simulink model "untitled"  (R2023b)
settings: Solver=VariableStepAuto  StartTime=0.0  StopTime=5  FixedStep=0.001  RelTol=1e-3
values from neighbouring files (symbols this model uses):
  i_a_rated = 27    [speed_control_by_field_weakening_parameter.m]
  J = 0.068    [speed_control_by_field_weakening_parameter.m]
  Ka = 1    [speed_control_by_field_weakening_parameter.m]
  La = 2.3e-3    (= 0.0023)    [speed_control_by_field_weakening_parameter.m]
  Ra = 0.3    [speed_control_by_field_weakening_parameter.m]
  speed_base = 2500*2*pi/60    (= 261.799387799)    [speed_control_by_field_weakening_parameter.m]
  speed_ref = 4500    [speed_control_by_field_weakening_parameter.m]
  Tload = 0    [speed_control_by_field_weakening_parameter.m]
  v_t_rated = 230    [speed_control_by_field_weakening_parameter.m]
libraries: slpidlib x2, simulink_extras x1
settings Model: NumberOfSteps=10  Creator=chayutht  LastModifiedBy=chayutht

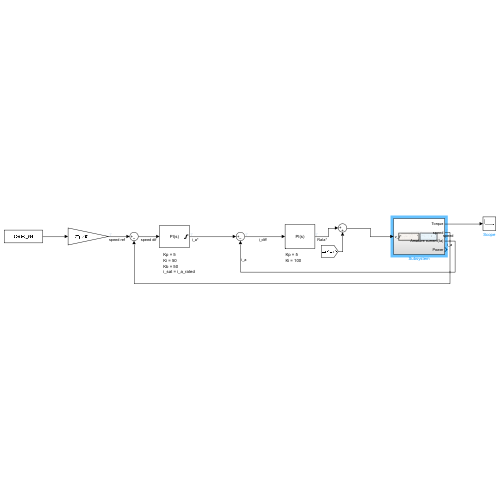
[thumbnail: Simulink's stored preview of the top-level diagram]
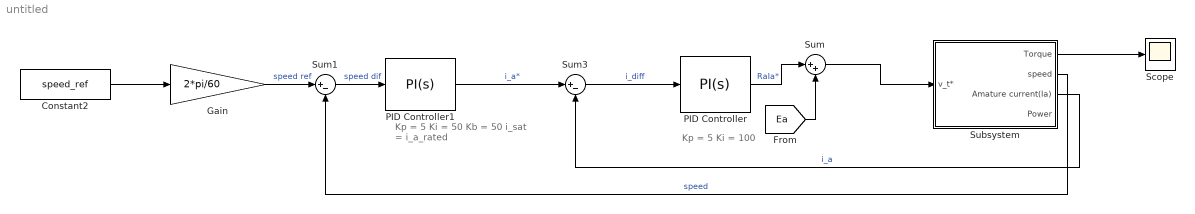
== system untitled ==
  note: Kp = 5
      | Ki = 100
  note: Kp = 5
      | Ki = 50
      | Kb = 50
      | i_sat = i_a_rated
  Constant2 : Constant  Value=speed_ref
  Gain : Gain  Gain=2*pi/60
  PID Controller : slpidlib/PID Controller  Controller=PI  Form=Parallel  TimeDomain=Continuous-time  UseExternalTs=off  SampleTime=-1  IntegratorMethod=Forward Euler  FilterMethod=Forward Euler  ControllerParametersSource=internal  P=5  I=100  UseKiTs=off  D=0.0001  N=100  UseFilter=on  TunerSelectOption=Frequency Response Based  InitialConditionSource=internal  InitialConditionForIntegrator=0  InitialConditionForFilter=0  DifferentiatorICPrevScaledInput=0  ExternalReset=none  TrackingMode=off  Kt=1  LimitOutput=off  SatLimitsSource=internal  UpperSaturationLimit=v_t_rated  LowerSaturationLimit=0  LinearizeAsGain=on  AntiWindupMode=none  Kb=1  LimitIntegrator=off  UpperIntegratorSaturationLimit=inf  LowerIntegratorSaturationLimit=-inf  POutMin=[]  POutMax=[]  IOutMin=[]  IOutMax=[]  DOutMin=[]  DOutMax=[]  NOutMin=[]  NOutMax=[]  SumOutMin=[]  SumOutMax=[]  SaturationOutMin=[]  SaturationOutMax=[]  PParamMin=[]  PParamMax=[]  IParamMin=[]  IParamMax=[]  DParamMin=[]  DParamMax=[]  NParamMin=[]  NParamMax=[]  KbParamMin=[]  KbParamMax=[]  KtParamMin=[]  KtParamMax=[]  KbOutMin=[]  KbOutMax=[]  KtOutMin=[]  KtOutMax=[]  IntegratorOutMin=[]  IntegratorOutMax=[]  FilterOutMin=[]  FilterOutMax=[]  SumI1OutMin=[]  SumI1OutMax=[]  SumI2OutMin=[]  SumI2OutMax=[]  SumI3OutMin=[]  SumI3OutMax=[]  SumI4OutMin=[]  SumI4OutMax=[]  SumDOutMin=[]  SumDOutMax=[]  DifferentiatorOutMin=[]  DifferentiatorOutMax=[]  FilterDiffOutCoefMin=[]  FilterDiffOutCoefMax=[]  ReciprocalOutMin=[]  ReciprocalOutMax=[]  SumDenOutMin=[]  SumDenOutMax=[]  SumNumOutMin=[]  SumNumOutMax=[]  DivideOutMin=[]  DivideOutMax=[]  UdiffTsProdOutMin=[]  UdiffTsProdOutMax=[]  NTsProdOutMin=[]  NTsProdOutMax=[]  UintegralTsProdOutMin=[]  UintegralTsProdOutMax=[]  UngainTsProdOutMin=[]  UngainTsProdOutMax=[]  ClampingZeroOutDataTypeStr=Inherit: Inherit via back propagation  ClampingZeroOutMin=[]  ClampingZeroOutMax=[]  FilterDenConstantOutDataTypeStr=Inherit: Inherit via back propagation  FilterDenConstantOutMin=[]  FilterDenConstantOutMax=[]  PCopyOutDataTypeStr=Inherit: Inherit via back propagation  PCopyOutMin=[]  PCopyOutMax=[]  NCopyOutDataTypeStr=Inherit: Inherit via back propagation  NCopyOutMin=[]  NCopyOutMax=[]  IntegratorContinuousStateAttributes=''  IntegratorStateMustResolveToSignalObject=off  IntegratorRTWStateStorageClass=Auto  FilterContinuousStateAttributes=''  FilterStateMustResolveToSignalObject=off  FilterRTWStateStorageClass=Auto  ParallelPVariant=InternalParameters  IdealPVariant=Disabled  IVariant=InternalParameters  DVariant=Disabled  IntegratorVariant=Continuous  SatVariant=Disabled  AWVariant=Passthrough  PCopyVariant=Disabled  TRVariant=Disabled  FdbkBlocksVariant=Forward  IdealPFdbkVariant=Disabled  SatFdbkVariant=Disabled  DerivativeFilterVariant=Disabled  NVariant=Disabled  NCopyVariant=Disabled_SignalSpec  FilterICVariant=Disabled  IntegratorICVariant=InternalICs  ExternalResetVariant=Disabled  TRSumVariant=Passthrough  SumFdbkVariant=Disabled  SumVariant=Sum_PI  TsampFilterVariant=InternalTs  TsampNgainVariant=Passthrough  TsampIntegralVariant=Disabled_SignalSpec  ExternalSaturationOutDataTypeStr=Inherit: Same as second input
  PID Controller1 : slpidlib/PID Controller  Controller=PI  Form=Parallel  TimeDomain=Continuous-time  UseExternalTs=off  SampleTime=-1  IntegratorMethod=Forward Euler  FilterMethod=Forward Euler  ControllerParametersSource=internal  P=5  I=50  UseKiTs=off  D=0.01  N=100  UseFilter=on  TunerSelectOption=Frequency Response Based  InitialConditionSource=internal  InitialConditionForIntegrator=0  InitialConditionForFilter=0  DifferentiatorICPrevScaledInput=0  ExternalReset=none  TrackingMode=off  Kt=1  LimitOutput=on  SatLimitsSource=internal  UpperSaturationLimit=i_a_rated  LowerSaturationLimit=-i_a_rated  LinearizeAsGain=on  AntiWindupMode=back-calculation  Kb=50  LimitIntegrator=off  UpperIntegratorSaturationLimit=inf  LowerIntegratorSaturationLimit=-inf  POutMin=[]  POutMax=[]  IOutMin=[]  IOutMax=[]  DOutMin=[]  DOutMax=[]  NOutMin=[]  NOutMax=[]  SumOutMin=[]  SumOutMax=[]  SaturationOutMin=[]  SaturationOutMax=[]  PParamMin=[]  PParamMax=[]  IParamMin=[]  IParamMax=[]  DParamMin=[]  DParamMax=[]  NParamMin=[]  NParamMax=[]  KbParamMin=[]  KbParamMax=[]  KtParamMin=[]  KtParamMax=[]  KbOutMin=[]  KbOutMax=[]  KtOutMin=[]  KtOutMax=[]  IntegratorOutMin=[]  IntegratorOutMax=[]  FilterOutMin=[]  FilterOutMax=[]  SumI1OutMin=[]  SumI1OutMax=[]  SumI2OutMin=[]  SumI2OutMax=[]  SumI3OutMin=[]  SumI3OutMax=[]  SumI4OutMin=[]  SumI4OutMax=[]  SumDOutMin=[]  SumDOutMax=[]  DifferentiatorOutMin=[]  DifferentiatorOutMax=[]  FilterDiffOutCoefMin=[]  FilterDiffOutCoefMax=[]  ReciprocalOutMin=[]  ReciprocalOutMax=[]  SumDenOutMin=[]  SumDenOutMax=[]  SumNumOutMin=[]  SumNumOutMax=[]  DivideOutMin=[]  DivideOutMax=[]  UdiffTsProdOutMin=[]  UdiffTsProdOutMax=[]  NTsProdOutMin=[]  NTsProdOutMax=[]  UintegralTsProdOutMin=[]  UintegralTsProdOutMax=[]  UngainTsProdOutMin=[]  UngainTsProdOutMax=[]  ClampingZeroOutDataTypeStr=Inherit: Inherit via back propagation  ClampingZeroOutMin=[]  ClampingZeroOutMax=[]  FilterDenConstantOutDataTypeStr=Inherit: Inherit via back propagation  FilterDenConstantOutMin=[]  FilterDenConstantOutMax=[]  PCopyOutDataTypeStr=Inherit: Inherit via back propagation  PCopyOutMin=[]  PCopyOutMax=[]  NCopyOutDataTypeStr=Inherit: Inherit via back propagation  NCopyOutMin=[]  NCopyOutMax=[]  IntegratorContinuousStateAttributes=''  IntegratorStateMustResolveToSignalObject=off  IntegratorRTWStateStorageClass=Auto  FilterContinuousStateAttributes=''  FilterStateMustResolveToSignalObject=off  FilterRTWStateStorageClass=Auto  ParallelPVariant=InternalParameters  IdealPVariant=Disabled  IVariant=InternalParameters  DVariant=Disabled  IntegratorVariant=Continuous  SatVariant=Enabled  AWVariant=BackCalculation  PCopyVariant=Disabled  TRVariant=Disabled  FdbkBlocksVariant=Forward  IdealPFdbkVariant=Disabled  SatFdbkVariant=Disabled  DerivativeFilterVariant=Disabled  NVariant=Disabled  NCopyVariant=Disabled_SignalSpec  FilterICVariant=Disabled  IntegratorICVariant=InternalICs  ExternalResetVariant=Disabled  TRSumVariant=Passthrough  SumFdbkVariant=Disabled  SumVariant=Sum_PI  TsampFilterVariant=InternalTs  TsampNgainVariant=Passthrough  TsampIntegralVariant=Disabled_SignalSpec  ExternalSaturationOutDataTypeStr=Inherit: Same as second input
  Scope : Scope
  Subsystem : Subsystem
  Sum : Sum  Inputs=|++
  Sum1 : Sum  Inputs=|+-
  Sum3 : Sum  Inputs=|+-
  wires:
  Subsystem/3(Amature current(Ia)) -> Sum3/2  "i_a"
  Subsystem/2(speed) -> Sum1/2  "speed"
  Subsystem/1(Torque) -> Scope/1
  Sum3/1 -> PID Controller/1  "i_diff"
  Sum1/1 -> PID Controller1/1  "speed dif"
  Constant2/1 -> Gain/1
  Gain/1 -> Sum1/1  "speed ref"
  PID Controller/1 -> Sum/1  "RaIa*"
  Sum/1 -> Subsystem/1(v_t*)
  [Ea] -> Sum/2
  PID Controller1/1 -> Sum3/1  "i_a*"

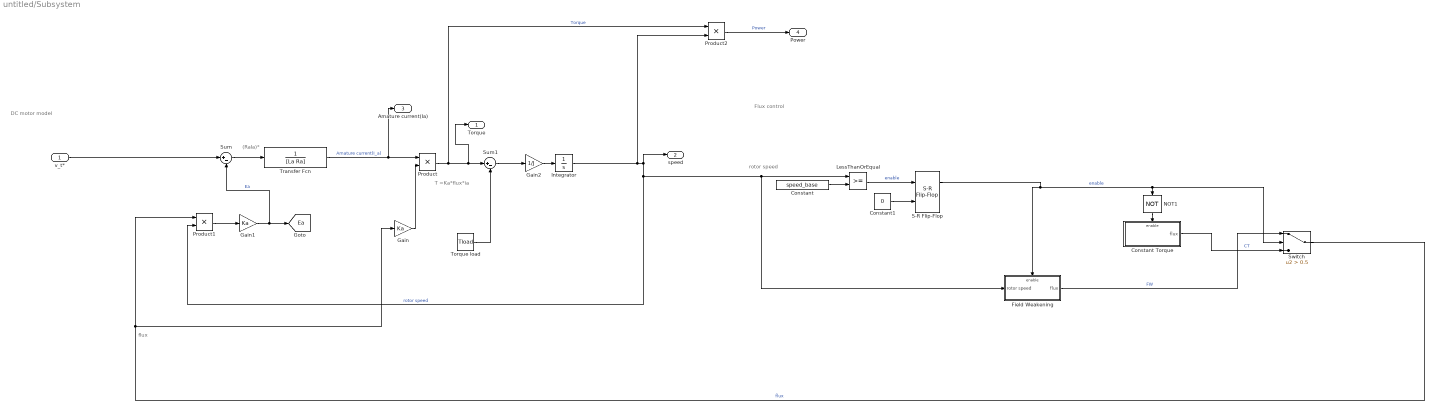
== system untitled/Subsystem ==
  note: rotor speed
  note: flux
  note: Flux control
  note: DC motor model
  note: (RaIa)*
  note: T =Ka*flux*ia
  v_t* : Inport
  Constant : Constant  Value=speed_base
  Constant Torque : Subsystem  TreatAsAtomicUnit=on
  Constant1 : Constant  Value=0  OutDataTypeStr=Inherit: Inherit via back propagation
  Field Weakening : Subsystem  TreatAsAtomicUnit=on
  Gain : Gain  Gain=Ka
  Gain1 : Gain  Gain=Ka
  Gain2 : Gain  Gain=1/J
  Integrator : Integrator
  LessThanOrEqual : RelationalOperator  OutDataTypeStr=boolean  RndMeth=Simplest  InputSameDT=off
  NOT1 : Logic  Operator=NOT  IconShape=distinctive  AllPortsSameDT=off  OutDataTypeStr=boolean
  Product : Product
  Product1 : Product
  Product2 : Product
  S-R Flip-Flop : simulink_extras/Flip Flops/S-R Flip-Flop  initial_condition=0
  Sum : Sum  Inputs=|+-
  Sum1 : Sum  Inputs=|+-
  Switch : Switch  Criteria=u2 > Threshold  Threshold=0.5  SaturateOnIntegerOverflow=off  InputSameDT=off
  Torque load : Constant  Value=Tload
  Transfer Fcn : TransferFcn  Denominator=[La Ra]
      settings: AttributesFormatString=%<Denominator>=(0.0023 0.3)
  Torque : Outport
  speed : Outport  Port=2
  Amature current(Ia) : Outport  Port=3
  Power : Outport  Port=4
  tag scope: Ea=global
  wires:
  Gain/1 -> Product/2
  Integrator/1 -> Product2/2, speed/1, Product1/2, Field Weakening/1(rotor speed), LessThanOrEqual/1  "rotor speed"
  Torque load/1 -> Sum1/2
  Sum1/1 -> Gain2/1
  v_t*/1 -> Sum/1
  Product/1 -> Product2/1, Sum1/1, Torque/1  "Torque"
  Gain2/1 -> Integrator/1
  Gain1/1 -> Sum/2, [Ea]  "Ea"
  Product1/1 -> Gain1/1
  Transfer Fcn/1 -> Amature current(Ia)/1, Product/1  "Amature current(I_a)"
  Sum/1 -> Transfer Fcn/1
  Switch/1 -> Gain/1, Product1/1  "flux"
  Constant/1 -> LessThanOrEqual/2
  Constant Torque/1(flux) -> Switch/3  "CT"
  S-R Flip-Flop/1 -> Field Weakening/Enable, NOT1/1, Switch/2  "enable"
  Field Weakening/1(flux) -> Switch/1  "FW"
  LessThanOrEqual/1 -> S-R Flip-Flop/1  "enable"
  NOT1/1 -> Constant Torque/Enable
  Constant1/1 -> S-R Flip-Flop/2
  Product2/1 -> Power/1  "Power"

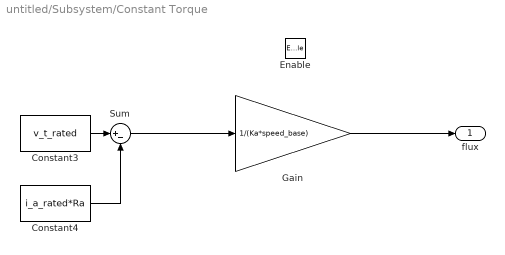
== system untitled/Subsystem/Constant Torque ==
  Enable : EnablePort
  Constant3 : Constant  Value=v_t_rated
  Constant4 : Constant  Value=i_a_rated*Ra
  Gain : Gain  Gain=1/(Ka*speed_base)
  Sum : Sum  Inputs=|+-
  flux : Outport
  wires:
  Gain/1 -> flux/1
  Constant3/1 -> Sum/1
  Constant4/1 -> Sum/2
  Sum/1 -> Gain/1

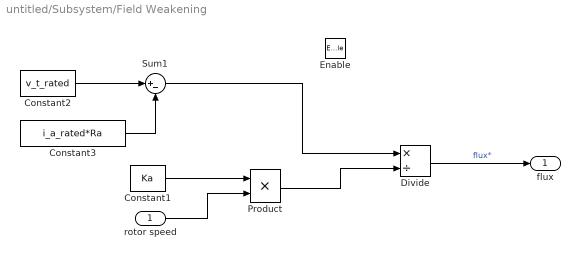
== system untitled/Subsystem/Field Weakening ==
  rotor speed : Inport
  Enable : EnablePort
  Constant1 : Constant  Value=Ka
  Constant2 : Constant  Value=v_t_rated
  Constant3 : Constant  Value=i_a_rated*Ra
  Divide : Product  Inputs=*/
  Product : Product
  Sum1 : Sum  Inputs=|+-
  flux : Outport
  wires:
  Constant1/1 -> Product/1
  rotor speed/1 -> Product/2
  Product/1 -> Divide/2
  Divide/1 -> flux/1  "flux*"
  Constant2/1 -> Sum1/1
  Constant3/1 -> Sum1/2
  Sum1/1 -> Divide/1
